simulink model "circuito_base"  (R2024b)
settings: Solver=VariableStepAuto  StartTime=0.0  StopTime=1048.0  RelTol=1e-3
values from neighbouring files (symbols this model uses):
  alpha = p(2)    [tclabsim.m]
  tau = p(3)    [tclabsim.m]
  U = p(1)    [tclabsim.m]
  x0 = x0 +273.15    [tclabsim.m]
settings Model: Creator=Hugo  LastModifiedBy=Hugo

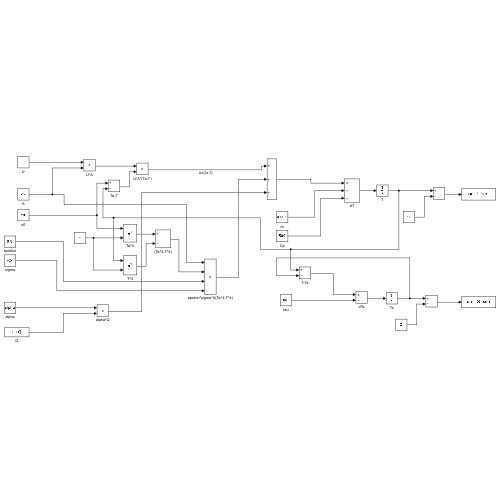
[thumbnail: Simulink's stored preview of the top-level diagram]
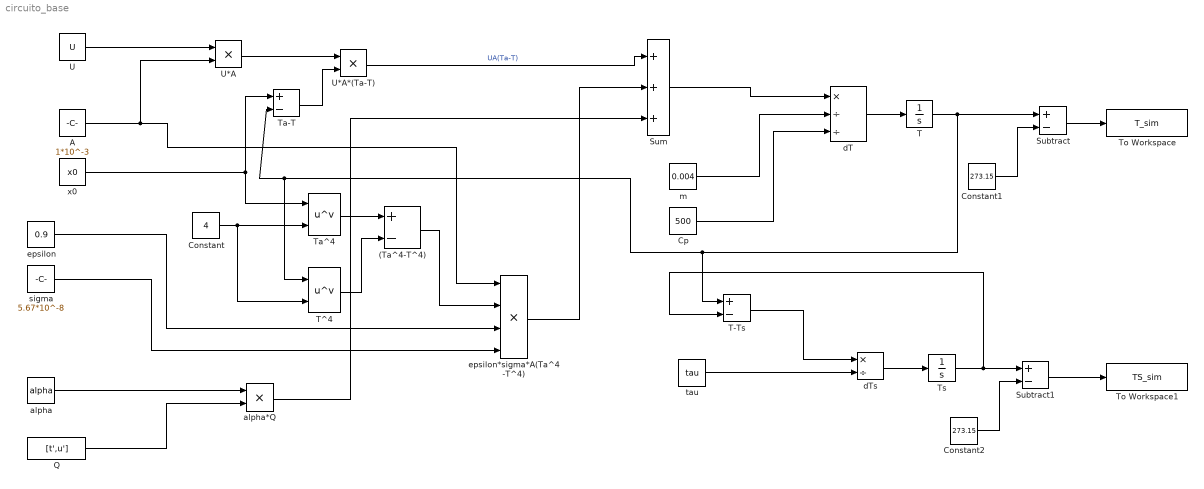
== system circuito_base ==
  (Ta^4-T^4) : Sum  Inputs=+-
  A : Constant  Value=1*10^-3
  Constant : Constant  Value=4
  Constant1 : Constant  Value=273.15
  Constant2 : Constant  Value=273.15
  Cp : Constant  Value=500
  Q : FromWorkspace  VariableName=[t',u']  SampleTime=2
  Subtract : Sum  Inputs=+-
  Subtract1 : Sum  Inputs=+-
  Sum : Sum  Inputs=+++
  T : Integrator  InitialCondition=x0
  T-Ts : Sum  Inputs=+-
  T^4 : Math  Operator=pow
  Ta-T : Sum  Inputs=+-
  Ta^4 : Math  Operator=pow
  To Workspace : ToWorkspace  VariableName=T_sim  SampleTime=2
  To Workspace1 : ToWorkspace  VariableName=TS_sim  SampleTime=2
  Ts : Integrator  InitialCondition=x0
  U : Constant  Value=U
  U*A : Product
  U*A*(Ta-T) : Product
  alpha : Constant  Value=alpha
  alpha*Q : Product
  dT : Product  Inputs=*//
  dTs : Product  Inputs=*/
  epsilon : Constant  Value=0.9
  epsilon*sigma*A(Ta^4-T^4) : Product  Inputs=4
  m : Constant  Value=0.004
  sigma : Constant  Value=5.67*10^-8
  tau : Constant  Value=tau
  x0 : Constant  Value=x0
  wires:
  U/1 -> U*A/1
  A/1 -> epsilon*sigma*A(Ta^4-T^4)/1, U*A/2
  U*A/1 -> U*A*(Ta-T)/1
  x0/1 -> Ta^4/1, Ta-T/1
  Ta-T/1 -> U*A*(Ta-T)/2
  Sum/1 -> dT/1
  U*A*(Ta-T)/1 -> Sum/1  "UA(Ta-T)"
  sigma/1 -> epsilon*sigma*A(Ta^4-T^4)/4
  Constant/1 -> T^4/2, Ta^4/2
  Ta^4/1 -> (Ta^4-T^4)/1
  T^4/1 -> (Ta^4-T^4)/2
  alpha/1 -> alpha*Q/1
  Q/1 -> alpha*Q/2
  m/1 -> dT/2
  Cp/1 -> dT/3
  dT/1 -> T/1
  T/1 -> Subtract/1, T-Ts/1, T^4/1, Ta-T/2
  Constant1/1 -> Subtract/2
  Subtract/1 -> To Workspace/1
  tau/1 -> dTs/2
  Subtract1/1 -> To Workspace1/1
  T-Ts/1 -> dTs/1
  dTs/1 -> Ts/1
  Ts/1 -> T-Ts/2, Subtract1/1
  Constant2/1 -> Subtract1/2
  epsilon/1 -> epsilon*sigma*A(Ta^4-T^4)/3
  (Ta^4-T^4)/1 -> epsilon*sigma*A(Ta^4-T^4)/2
  epsilon*sigma*A(Ta^4-T^4)/1 -> Sum/2
  alpha*Q/1 -> Sum/3
